simulink model "Outer_Loop_Autopilot"  (R2021b)
settings: Solver=FixedStepAuto  StartTime=0.0  StopTime=10.0  FixedStep=0.01  RelTol=1e-3
model workspace (MAT data in the model file):
  airspeedVal = 36.8390748719
  lastWaypointInstance = [-1135.6394405; 2105.53264134; -191.7192]
  waypointData = [-134.018235705 -135.221787528 -136.425541281 -137.629496916 -138.83365438 -140.038013624 -141.242574597 -142.447337247 -143.652301524 -144.857467378 -146.062966192 -147.268871083 ... (2697 elements, 899x3)]
undefined symbols (not defined in the file): ap, uavParam
libraries: slpidlib x4, simulink x3, slctrlblks x1, simulink_need_slupdate x1
(part 1 of 2)
settings Model: DataDictionary=stepFideltyResponseData.sldd  ModifiedByFormat=The MathWorks, Inc.  Creator=The MathWorks, Inc.  LastModifiedBy=The MathWorks, Inc.
settings DataIOCC: SaveOutput=off  SaveTime=off
settings OptimizationCC: UseDivisionForNetSlopeComputation=UseDivisionForReciprocalsOfIntegersOnly

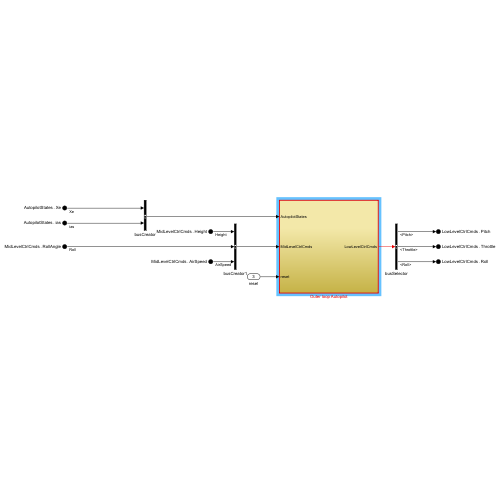
[thumbnail: Simulink's stored preview of the top-level diagram]
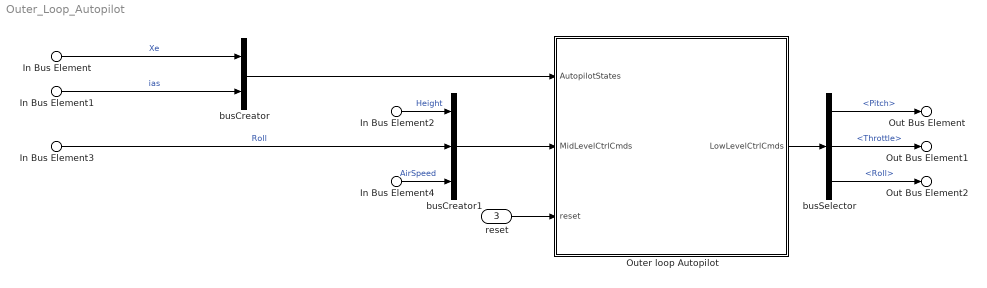
== system Outer_Loop_Autopilot ==
  In Bus Element : Inport  PortName=AutopilotStates  Element=Xe
  In Bus Element1 : Inport  PortName=AutopilotStates  Element=ias
  In Bus Element2 : Inport  Port=2  PortName=MidLevelCtrlCmds  Element=Height
  In Bus Element3 : Inport  Port=2  PortName=MidLevelCtrlCmds  Element=RollAngle
  In Bus Element4 : Inport  Port=2  PortName=MidLevelCtrlCmds  Element=AirSpeed
  reset : Inport  Port=3  OutDataTypeStr=double  PortDimensions=1  SampleTime=[0.01,0]
  Outer loop Autopilot : Subsystem  TreatAsAtomicUnit=on
  busCreator : BusCreator  Inputs=2
  busCreator1 : BusCreator  Inputs=3
  busSelector : BusSelector  OutputSignals=Pitch,Throttle,Roll
  Out Bus Element : Outport  PortName=LowLevelCtrlCmds  Element=Pitch
  Out Bus Element1 : Outport  PortName=LowLevelCtrlCmds  Element=Throttle
  Out Bus Element2 : Outport  PortName=LowLevelCtrlCmds  Element=Roll
  wires:
  busCreator1/1 -> Outer loop Autopilot/2(MidLevelCtrlCmds)
  Outer loop Autopilot/1(LowLevelCtrlCmds) -> busSelector/1
  In Bus Element/1 -> busCreator/1  "Xe"
  In Bus Element4/1 -> busCreator1/3  "AirSpeed"
  In Bus Element2/1 -> busCreator1/1  "Height"
  reset/1 -> Outer loop Autopilot/3(reset)
  In Bus Element3/1 -> busCreator1/2  "Roll"
  busCreator/1 -> Outer loop Autopilot/1(AutopilotStates)
  busSelector/1 -> Out Bus Element/1  "<Pitch>"
  busSelector/2 -> Out Bus Element1/1  "<Throttle>"
  busSelector/3 -> Out Bus Element2/1  "<Roll>"
  In Bus Element1/1 -> busCreator/2  "ias"

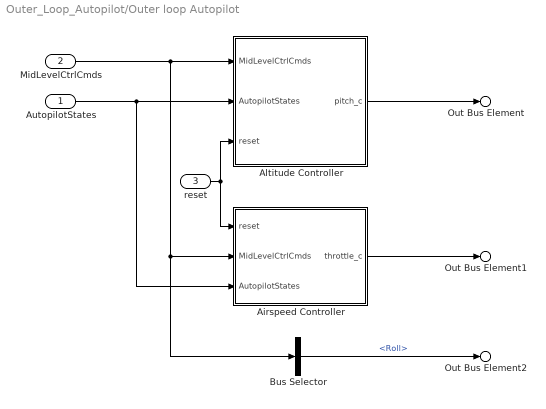
== system Outer_Loop_Autopilot/Outer loop Autopilot ==
  AutopilotStates : Inport
  MidLevelCtrlCmds : Inport  Port=2
  reset : Inport  Port=3
  Airspeed Controller : Subsystem  VariantControl=AirspeedCont~=1
  Altitude Controller : Subsystem  VariantControl=AltCont==0
  Bus Selector : BusSelector  OutputSignals=Roll
  Out Bus Element : Outport  PortName=LowLevelCtrlCmds  Element=Pitch
  Out Bus Element1 : Outport  PortName=LowLevelCtrlCmds  Element=Throttle
  Out Bus Element2 : Outport  PortName=LowLevelCtrlCmds  Element=Roll
  wires:
  Altitude Controller/1(pitch_c) -> Out Bus Element/1
  Airspeed Controller/1(throttle_c) -> Out Bus Element1/1
  Bus Selector/1 -> Out Bus Element2/1  "<Roll>"
  AutopilotStates/1 -> Altitude Controller/2(AutopilotStates), Airspeed Controller/3(AutopilotStates)
  MidLevelCtrlCmds/1 -> Airspeed Controller/2(MidLevelCtrlCmds), Bus Selector/1, Altitude Controller/1(MidLevelCtrlCmds)
  reset/1 -> Airspeed Controller/1(reset), Altitude Controller/3(reset)

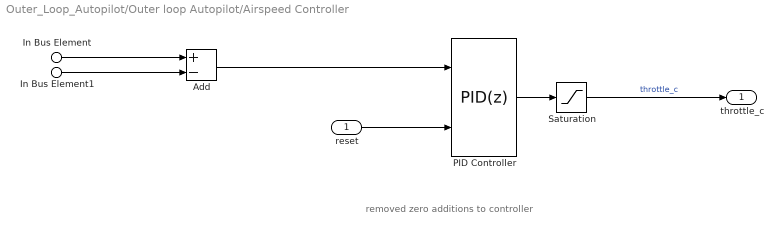
== system Outer_Loop_Autopilot/Outer loop Autopilot/Airspeed Controller ==
  note: removed zero additions to controller
  reset : Inport
  In Bus Element : Inport  Port=2  PortName=MidLevelCtrlCmds  Element=AirSpeed
  In Bus Element1 : Inport  Port=3  PortName=AutopilotStates  Element=ias
  Add : Sum  Inputs=+-
  PID Controller : slpidlib/PID Controller  Controller=PID  Form=Parallel  TimeDomain=Discrete-time  UseExternalTs=off  SampleTime=0.01  IntegratorMethod=Trapezoidal  FilterMethod=Forward Euler  ControllerParametersSource=internal  P=1.3  I=0.15  D=0.1  UseFilter=on  N=ap.control.derivativesConstant  TunerSelectOption=Transfer Function Based (PID Tuner App)  InitialConditionSource=internal  InitialConditionForIntegrator=0  InitialConditionForFilter=0  DifferentiatorICPrevScaledInput=0  ExternalReset=level  TrackingMode=off  Kt=1  LimitOutput=on  SatLimitsSource=internal  UpperSaturationLimit=ap.control.dtLimit  LowerSaturationLimit=0  LinearizeAsGain=on  AntiWindupMode=clamping  Kb=1  POutMin=[]  POutMax=[]  IOutMin=[]  IOutMax=[]  DOutMin=[]  DOutMax=[]  NOutMin=[]  NOutMax=[]  SumOutMin=[]  SumOutMax=[]  SaturationOutMin=[]  SaturationOutMax=[]  PParamMin=[]  PParamMax=[]  IParamMin=[]  IParamMax=[]  DParamMin=[]  DParamMax=[]  NParamMin=[]  NParamMax=[]  KbParamMin=[]  KbParamMax=[]  KtParamMin=[]  KtParamMax=[]  KbOutMin=[]  KbOutMax=[]  KtOutMin=[]  KtOutMax=[]  IntegratorOutMin=[]  IntegratorOutMax=[]  FilterOutMin=[]  FilterOutMax=[]  SumI1OutMin=[]  SumI1OutMax=[]  SumI2OutMin=[]  SumI2OutMax=[]  SumI3OutMin=[]  SumI3OutMax=[]  SumI4OutMin=[]  SumI4OutMax=[]  SumDOutMin=[]  SumDOutMax=[]  DifferentiatorOutMin=[]  DifferentiatorOutMax=[]  FilterDiffOutCoefMin=[]  FilterDiffOutCoefMax=[]  ReciprocalOutMin=[]  ReciprocalOutMax=[]  SumDenOutMin=[]  SumDenOutMax=[]  SumNumOutMin=[]  SumNumOutMax=[]  DivideOutMin=[]  DivideOutMax=[]  UdiffTsProdOutMin=[]  UdiffTsProdOutMax=[]  NTsProdOutMin=[]  NTsProdOutMax=[]  UintegralTsProdOutMin=[]  UintegralTsProdOutMax=[]  UngainTsProdOutMin=[]  UngainTsProdOutMax=[]  FilterDenConstantOutDataTypeStr=Inherit: Inherit via back propagation  FilterDenConstantOutMin=[]  FilterDenConstantOutMax=[]  PCopyOutDataTypeStr=Inherit: Inherit via back propagation  PCopyOutMin=[]  PCopyOutMax=[]  NCopyOutDataTypeStr=Inherit: Inherit via back propagation  NCopyOutMin=[]  NCopyOutMax=[]  IntegratorContinuousStateAttributes=''  IntegratorStateMustResolveToSignalObject=off  IntegratorRTWStateStorageClass=Auto  FilterContinuousStateAttributes=''  FilterStateMustResolveToSignalObject=off  FilterRTWStateStorageClass=Auto  ParallelPVariant=InternalParameters  IdealPVariant=Disabled  IVariant=InternalParameters  DVariant=InternalParameters  IntegratorVariant=Discrete  SatVariant=Enabled  AWVariant=DiscClampingParallel  PCopyVariant=Disabled  TRVariant=Disabled  FdbkBlocksVariant=Feedback  IdealPFdbkVariant=Passthrough  SatFdbkVariant=Passthrough  DerivativeFilterVariant=ForwardEulerFilter  NVariant=InternalParameters  NCopyVariant=Disabled  FilterICVariant=InternalICsFilter  IntegratorICVariant=InternalICs  ExternalResetVariant=ExternalReset  TRSumVariant=Passthrough  SumFdbkVariant=Enabled  SumVariant=Sum_PID  TsampFilterVariant=InternalTs  TsampNgainVariant=Passthrough  TsampIntegralVariant=Passthrough  ExternalSaturationOutDataTypeStr=Inherit: Same as second input
  Saturation : Saturate  UpperLimit=ap.control.dtLimit  LowerLimit=0  OutDataTypeStr=double
  throttle_c : Outport
  wires:
  PID Controller/1 -> Saturation/1
  reset/1 -> PID Controller/2
  In Bus Element1/1 -> Add/2
  In Bus Element/1 -> Add/1
  Saturation/1 -> throttle_c/1  "throttle_c"
  Add/1 -> PID Controller/1

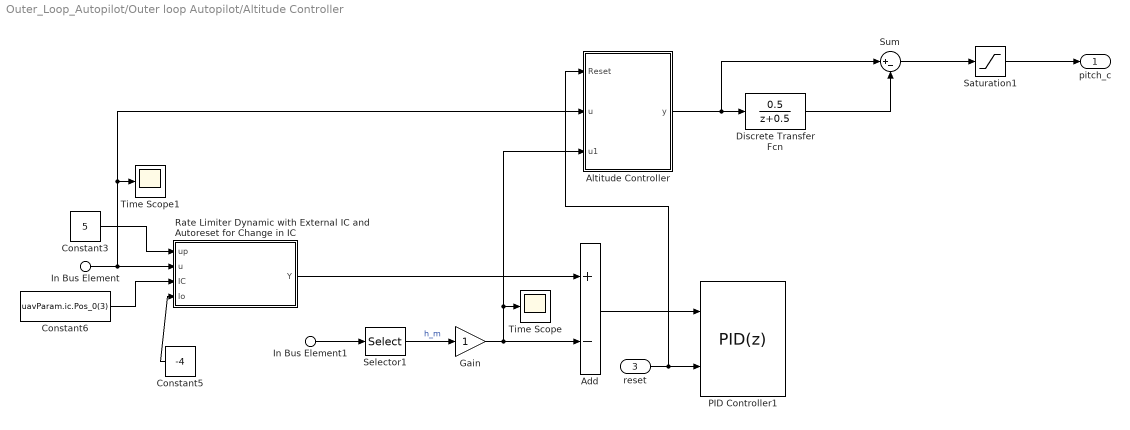
== system Outer_Loop_Autopilot/Outer loop Autopilot/Altitude Controller ==
  In Bus Element : Inport  PortName=MidLevelCtrlCmds  Element=Height
  In Bus Element1 : Inport  Port=2  PortName=AutopilotStates  Element=Xe
  reset : Inport  Port=3
  Add : Sum  Inputs=+-
  Altitude Controller : Subsystem
  Constant3 : Constant  Value=5  OutDataTypeStr=Inherit: Inherit via back propagation
      settings: AttributesFormatString=%<Value>
  Constant5 : Constant  Value=-4  OutDataTypeStr=Inherit: Inherit via back propagation
      settings: AttributesFormatString=%<Value>
  Constant6 : Constant  Value=uavParam.ic.Pos_0(3)  OutDataTypeStr=double
      settings: AttributesFormatString=%<Value>
  Discrete Transfer Fcn : DiscreteTransferFcn  Numerator=[0.5]
  Gain : Gain
  PID Controller1 : slpidlib/PID Controller  Controller=PID  Form=Parallel  TimeDomain=Discrete-time  UseExternalTs=off  SampleTime=0.01  IntegratorMethod=Trapezoidal  FilterMethod=Forward Euler  ControllerParametersSource=internal  P=1.3  I=5  D=.5  UseFilter=off  N=5  TunerSelectOption=Frequency Response Based  InitialConditionSource=internal  InitialConditionForIntegrator=0  InitialConditionForFilter=0  DifferentiatorICPrevScaledInput=0  ExternalReset=level  TrackingMode=off  Kt=1  LimitOutput=on  SatLimitsSource=internal  UpperSaturationLimit=ap.control.the_cLimit  LowerSaturationLimit=-ap.control.the_cLimit  LinearizeAsGain=on  AntiWindupMode=clamping  Kb=1  POutMin=[]  POutMax=[]  IOutMin=[]  IOutMax=[]  DOutMin=[]  DOutMax=[]  NOutMin=[]  NOutMax=[]  SumOutMin=[]  SumOutMax=[]  SaturationOutMin=[]  SaturationOutMax=[]  PParamMin=[]  PParamMax=[]  IParamMin=[]  IParamMax=[]  DParamMin=[]  DParamMax=[]  NParamMin=[]  NParamMax=[]  KbParamMin=[]  KbParamMax=[]  KtParamMin=[]  KtParamMax=[]  KbOutMin=[]  KbOutMax=[]  KtOutMin=[]  KtOutMax=[]  IntegratorOutMin=[]  IntegratorOutMax=[]  FilterOutMin=[]  FilterOutMax=[]  SumI1OutMin=[]  SumI1OutMax=[]  SumI2OutMin=[]  SumI2OutMax=[]  SumI3OutMin=[]  SumI3OutMax=[]  SumI4OutMin=[]  SumI4OutMax=[]  SumDOutMin=[]  SumDOutMax=[]  DifferentiatorOutMin=[]  DifferentiatorOutMax=[]  FilterDiffOutCoefMin=[]  FilterDiffOutCoefMax=[]  ReciprocalOutMin=[]  ReciprocalOutMax=[]  SumDenOutMin=[]  SumDenOutMax=[]  SumNumOutMin=[]  SumNumOutMax=[]  DivideOutMin=[]  DivideOutMax=[]  UdiffTsProdOutMin=[]  UdiffTsProdOutMax=[]  NTsProdOutMin=[]  NTsProdOutMax=[]  UintegralTsProdOutMin=[]  UintegralTsProdOutMax=[]  UngainTsProdOutMin=[]  UngainTsProdOutMax=[]  FilterDenConstantOutDataTypeStr=Inherit: Inherit via back propagation  FilterDenConstantOutMin=[]  FilterDenConstantOutMax=[]  PCopyOutDataTypeStr=Inherit: Inherit via back propagation  PCopyOutMin=[]  PCopyOutMax=[]  NCopyOutDataTypeStr=Inherit: Inherit via back propagation  NCopyOutMin=[]  NCopyOutMax=[]  IntegratorContinuousStateAttributes=''  IntegratorStateMustResolveToSignalObject=off  IntegratorRTWStateStorageClass=Auto  FilterContinuousStateAttributes=''  FilterStateMustResolveToSignalObject=off  FilterRTWStateStorageClass=Auto  ParallelPVariant=InternalParameters  IdealPVariant=Disabled  IVariant=InternalParameters  DVariant=InternalParameters  IntegratorVariant=Discrete  SatVariant=Enabled  AWVariant=DiscClampingParallel  PCopyVariant=Disabled  TRVariant=Disabled  FdbkBlocksVariant=Feedback  IdealPFdbkVariant=Passthrough  SatFdbkVariant=Passthrough  DerivativeFilterVariant=Differentiator  NVariant=Passthrough  NCopyVariant=Disabled_SignalSpec  FilterICVariant=InternalICsDifferentiator  IntegratorICVariant=InternalICs  ExternalResetVariant=ExternalReset  TRSumVariant=Passthrough  SumFdbkVariant=Enabled  SumVariant=Sum_PID  TsampFilterVariant=InternalTs  TsampNgainVariant=Passthrough  TsampIntegralVariant=Passthrough  ExternalSaturationOutDataTypeStr=Inherit: Same as second input
  Rate Limiter Dynamic with External IC and Autoreset for Change in IC : Subsystem
      mask Display:
      | plot([0.15 0.95],[.5 .5],[.5 .5],[0.05 0.95],0.05+0.9*[.2 .8],0.05+0.9*[0 1]);
      | port_label('output',1,'Y');
      | port_label('input',1,'up');
      | port_label('input',2,'u');
      | port_label('input',3,'IC');
      | port_label('input',4,'Lo');
  Saturation1 : Saturate  UpperLimit=ap.control.the_cLimit  LowerLimit=-ap.control.the_cLimit  OutDataTypeStr=double
  Selector1 : Selector  InputPortWidth=3  IndexOptions=Index vector (dialog)  Indices=[3]  OutputSizes=1
  Sum : Sum  Inputs=|+-
  Time Scope : Scope
  Time Scope1 : Scope
  pitch_c : Outport
  wires:
  Selector1/1 -> Gain/1  "h_m"
  Rate Limiter Dynamic with External IC and Autoreset for Change in IC/1(Y) -> Add/1
  Add/1 -> PID Controller1/1
  Constant6/1 -> Rate Limiter Dynamic with External IC and Autoreset for Change in IC/3(IC)
  Constant3/1 -> Rate Limiter Dynamic with External IC and Autoreset for Change in IC/1(up)
  Constant5/1 -> Rate Limiter Dynamic with External IC and Autoreset for Change in IC/4(lo)
  In Bus Element1/1 -> Selector1/1
  Gain/1 -> Altitude Controller/3(u1), Time Scope/1, Add/2
  Saturation1/1 -> pitch_c/1
  reset/1 -> Altitude Controller/1(Reset), PID Controller1/2
  Discrete Transfer Fcn/1 -> Sum/2
  Sum/1 -> Saturation1/1
  Altitude Controller/1(y) -> Sum/1, Discrete Transfer Fcn/1
  In Bus Element/1 -> Altitude Controller/2(u), Time Scope1/1, Rate Limiter Dynamic with External IC and Autoreset for Change in IC/2(u)
